simulink model "VMC_14Dof_2024a"  (R2024a)
settings: Solver=FixedStepDiscrete  StartTime=0.0  StopTime=10.0  FixedStep=0.001  RelTol=1e-3
InitFcn:
  | unlinear_14DOF_Parameters
undefined symbols (not defined in the file): Bf, Br, Cp_fl, Cp_fr, Cp_rl, Cp_rr, Cs_f, eta_FMotor, eta_RMotor, f, g, He, Hp, i_fa, i_ra, i_sw, I_tire, Ix, Iy, Iz, ks_f, kw, Lf, Lr, m, mb, mu, mw, r, Sampletime, Standstill_buffer, vx0, vxlim, w0
libraries: simulink x32, slpidlib x6
(part 3 of 5)

== system VMC_14Dof_2024a/Subsystem1/Vehicle_State_Estimation/Steering_Angle ==
  SteeringWheelAngle_deg : Inport
  Constant3 : Constant  Value=0  OutDataTypeStr=single  SampleTime=-1
  Constant4 : Constant  Value=0  OutDataTypeStr=single  SampleTime=-1
  FWA_FL_Table_deg : Lookup_n-D  NumberOfTableDimensions=1  BreakpointsForDimension1=|  BreakpointsForDimension1DataTypeStr=single  Table=|  TableDataTypeStr=single  IntermediateResultsDataTypeStr=single  InternalRulePriority=Speed  OutDataTypeStr=single  RndMeth=Simplest  FractionDataTypeStr=single
      BreakpointsForDimension1=|
      | [-117
      | -116
      | -115
      | -114
      | -113
      | -112
      | -111
      | -110
      | -109
      | -108
      | -107
      | -106
      | -105
      | -104
      | -103
      | -102
      | -101
      | -100
      | -99
      | -98
      | -97
      | -96
      | -95
      | -94
      | -93
      | -92
      | -91
      | -90
      | -89
      | -88
      | -87
      | -86
      | -85
      | -84
      | -83
      | -82
      | -81
      | -80
      | -79
      | -78
      | -77
      | -76
      | -75
      | -74
      | -73
      | -72
      | -71
      | -70
      | -69
      | -68
      | -67
      | -66
      | -65
      | -64
      | -63
      | -62
      | -61
      | -60
      | -59
      | -58
      | -57
      | -56
      | -55
      | -54
      | -53
      | -52
      | -51
      | -50
      | -49
      | -48
      | -47
      | -46
      | -45
      | -44
      | -43
      | -42
      | -41
      | -40
      | -39
      | -38
      | -37
      | -36
      | -35
      | -34
      | -33
      | -32
      | -31
      | -30
      | -29
      | -28
      | -27
      | -26
      | -25
      | -24
      | -23
      | -22
      | -21
      | -20
      | -19
      | -18
      | -17
      | -16
      | -15
      | -14
      | -13
      | -12
      | -11
      | -10
      | -9
      | -8
      | -7
      | -6
      | -5
      | -4
      | -3
      | -2
      | -1
      | 0
      | 1
      | 2
      | 3
      | 4
      | 5
      | 6
      | 7
      | 8
      | 9
      | 10
      | 11
      | 12
      | 13
      | 14
      | 15
      | 16
      | 17
      | 18
      | 19
      | 20
      | 21
      | 22
      | 23
      | 24
      | 25
      | 26
      | 27
      | 28
      | 29
      | 30
      | 31
      | 32
      | 33
      | 34
      | 35
      | 36
      | 37
      | 38
      | 39
      | 40
      | 41
      | 42
      | 43
      | 44
      | 45
      | 46
      | 47
      | 48
      | 49
      | 50
      | 51
      | 52
      | 53
      | 54
      | 55
      | 56
      | 57
      | 58
      | 59
      | 60
      | 61
      | 62
      | 63
      | 64
      | 65
      | 66
      | 67
      | 68
      | 69
      | 70
      | 71
      | 72
      | 73
      | 74
      | 75
      | 76
      | 77
      | 78
      | 79
      | 80
      | 81
      | 82
      | 83
      | 84
      | 85
      | 86
      | 87
      | 88
      | 89
      | 90
      | 91
      | 92
      | 93
      | 94
      | 95
      | 96
      | 97
      | 98
      | 99
      | 100
      | 101
      | 102
      | 103
      | 104
      | 105
      | 106
      | 107
      | 108
      | 109
      | 110
      | 111
      | 112
      | 113
      | 114
      | 115
      | 116
      | 117]
      Table=|
      | [-23.05316527
      | -22.85986982
      | -22.66659264
      | -22.47333151
      | -22.28008425
      | -22.08684866
      | -21.89362256
      | -21.70040379
      | -21.50719018
      | -21.31397955
      | -21.12076975
      | -20.92755864
      | -20.73434405
      | -20.54112386
      | -20.34789591
      | -20.15465809
      | -19.96140824
      | -19.76814426
      | -19.57486401
      | -19.38156538
      | -19.18824624
      | -18.99490448
      | -18.801538
      | -18.60814467
      | -18.4147224
      | -18.22126908
      | -18.0277826
      | -17.83426085
      | -17.64070175
      | -17.44710317
      | -17.25346304
      | -17.05977924
      | -16.86604968
      | -16.67227225
      | -16.47844486
      | -16.2845654
      | -16.09063178
      | -15.89664189
      | -15.70259363
      | -15.5084849
      | -15.31431358
      | -15.12007757
      | -14.92577477
      | -14.73140306
      | -14.53696032
      | -14.34244444
      | -14.14785329
      | -13.95318476
      | -13.75843671
      | -13.56360702
      | -13.36869356
      | -13.17369417
      | -12.97860673
      | -12.78342908
      | -12.58815908
      | -12.39279455
      | -12.19733335
      | -12.00177331
      | -11.80611224
      | -11.61034798
      | -11.41447833
      | -11.2185011
      | -11.0224141
      | -10.82621511
      | -10.62990193
      | -10.43347233
      | -10.23692409
      | -10.04025496
      | -9.843462713
      | -9.646545082
      | -9.449499809
      | -9.252324623
      | -9.055017243
      | -8.857575379
      | -8.659996732
      | -8.46227899
      | -8.264419833
      | -8.066416931
      | -7.868267939
      | -7.669970506
      | -7.471522265
      | -7.27292084
      | -7.07416384
      | -6.875248864
      | -6.676173498
      | -6.476935313
      | -6.277531868
      | -6.077960708
      | -5.878219363
      | -5.678305351
      | -5.478216172
      | -5.277949314
      | -5.077502247
      | -4.876872426
      | -4.676057291
      | -4.475054264
      | -4.273860752
      | -4.072474141
      | -3.870891803
      | -3.669111092
      | -3.467129341
      | -3.264943865
      | -3.062551963
      | -2.859950909
      | -2.657137961
      | -2.454110356
      | -2.250865308
      | -2.047400013
      | -1.843711642
      | -1.639797346
      | -1.435654252
      | -1.231279465
      | -1.026670065
      | -0.82182311
      | -0.616735632
      | -0.411404637
      | -0.205827108
      | 0
      | 0.206079759
      | 0.412415266
      | 0.619009648
      | 0.825866059
      | 1.032987682
      | 1.240377731
      | 1.448039447
      | 1.655976105
      | 1.864191008
      | 2.072687493
      | 2.28146893
      | 2.49053872
      | 2.6999003
      | 2.909557141
      | 3.119512748
      | 3.329770663
      | 3.540334465
      | 3.75120777
      | 3.962394233
      | 4.173897546
      | 4.385721443
      | 4.597869697
      | 4.810346123
      | 5.02315458
      | 5.236298967
      | 5.449783228
      | 5.663611355
      | 5.877787381
      | 6.09231539
      | 6.307199511
      | 6.522443924
      | 6.738052856
      | 6.954030589
      | 7.170381452
      | 7.387109832
      | 7.604220167
      | 7.821716951
      | 8.039604735
      | 8.257888127
      | 8.476571794
      | 8.695660466
      | 8.915158929
      | 9.135072038
      | 9.355404708
      | 9.576161921
      | 9.797348726
      | 10.01897024
      | 10.24103166
      | 10.46353823
      | 10.68649529
      | 10.90990825
      | 11.1337826
      | 11.35812389
      | 11.58293777
      | 11.80822996
      | 12.03400628
      | 12.26027261
      | 12.48703495
      | 12.71429936
      | 12.94207201
      | 13.17035916
      | 13.39916716
      | 13.62850247
      | 13.85837164
      | 14.08878133
      | 14.3197383
      | 14.55124944
      | 14.78332172
      | 15.01596225
      | 15.24917823
      | 15.48297702
      | 15.71736605
      | 15.95235293
      | 16.18794536
      | 16.42415119
      | 16.66097841
      | 16.89843513
      | 17.13652963
      | 17.3752703
      | 17.61466573
      | 17.85472462
      | 18.09545586
      | 18.33686848
      | 18.5789717
      | 18.82177488
      | 19.06528761
      | 19.3095196
      | 19.55448079
      | 19.80018131
      | 20.04663146
      | 20.29384178
      | 20.54182299
      | 20.79058604
      | 21.0401421
      | 21.29050257
      | 21.54167908
      | 21.79368351
      | 22.04652799
      | 22.3002249
      | 22.55478688
      | 22.81022687
      | 23.06655806
      | 23.32379396
      | 23.58194836
      | 23.84103537
      | 24.10106942
      | 24.36206527
      | 24.62403801
      | 24.88700311
      | 25.15097637
      | 25.415974
      | 25.68201259
      | 25.94910911
      | 26.217281
      | 26.48654607
      | 26.75692263
      | 27.02842943
      | ]
  FWA_FR_Table_deg : Lookup_n-D  NumberOfTableDimensions=1  BreakpointsForDimension1=|  BreakpointsForDimension1DataTypeStr=single  Table=|  TableDataTypeStr=single  IntermediateResultsDataTypeStr=single  InternalRulePriority=Speed  OutDataTypeStr=single  RndMeth=Simplest  FractionDataTypeStr=single
      BreakpointsForDimension1=|
      | [-117
      | -116
      | -115
      | -114
      | -113
      | -112
      | -111
      | -110
      | -109
      | -108
      | -107
      | -106
      | -105
      | -104
      | -103
      | -102
      | -101
      | -100
      | -99
      | -98
      | -97
      | -96
      | -95
      | -94
      | -93
      | -92
      | -91
      | -90
      | -89
      | -88
      | -87
      | -86
      | -85
      | -84
      | -83
      | -82
      | -81
      | -80
      | -79
      | -78
      | -77
      | -76
      | -75
      | -74
      | -73
      | -72
      | -71
      | -70
      | -69
      | -68
      | -67
      | -66
      | -65
      | -64
      | -63
      | -62
      | -61
      | -60
      | -59
      | -58
      | -57
      | -56
      | -55
      | -54
      | -53
      | -52
      | -51
      | -50
      | -49
      | -48
      | -47
      | -46
      | -45
      | -44
      | -43
      | -42
      | -41
      | -40
      | -39
      | -38
      | -37
      | -36
      | -35
      | -34
      | -33
      | -32
      | -31
      | -30
      | -29
      | -28
      | -27
      | -26
      | -25
      | -24
      | -23
      | -22
      | -21
      | -20
      | -19
      | -18
      | -17
      | -16
      | -15
      | -14
      | -13
      | -12
      | -11
      | -10
      | -9
      | -8
      | -7
      | -6
      | -5
      | -4
      | -3
      | -2
      | -1
      | 0
      | 1
      | 2
      | 3
      | 4
      | 5
      | 6
      | 7
      | 8
      | 9
      | 10
      | 11
      | 12
      | 13
      | 14
      | 15
      | 16
      | 17
      | 18
      | 19
      | 20
      | 21
      | 22
      | 23
      | 24
      | 25
      | 26
      | 27
      | 28
      | 29
      | 30
      | 31
      | 32
      | 33
      | 34
      | 35
      | 36
      | 37
      | 38
      | 39
      | 40
      | 41
      | 42
      | 43
      | 44
      | 45
      | 46
      | 47
      | 48
      | 49
      | 50
      | 51
      | 52
      | 53
      | 54
      | 55
      | 56
      | 57
      | 58
      | 59
      | 60
      | 61
      | 62
      | 63
      | 64
      | 65
      | 66
      | 67
      | 68
      | 69
      | 70
      | 71
      | 72
      | 73
      | 74
      | 75
      | 76
      | 77
      | 78
      | 79
      | 80
      | 81
      | 82
      | 83
      | 84
      | 85
      | 86
      | 87
      | 88
      | 89
      | 90
      | 91
      | 92
      | 93
      | 94
      | 95
      | 96
      | 97
      | 98
      | 99
      | 100
      | 101
      | 102
      | 103
      | 104
      | 105
      | 106
      | 107
      | 108
      | 109
      | 110
      | 111
      | 112
      | 113
      | 114
      | 115
      | 116
      | 117]
      Table=|
      | [-27.02842943
      | -26.75692263
      | -26.48654607
      | -26.217281
      | -25.94910911
      | -25.68201259
      | -25.415974
      | -25.15097637
      | -24.88700311
      | -24.62403801
      | -24.36206527
      | -24.10106942
      | -23.84103537
      | -23.58194836
      | -23.32379396
      | -23.06655806
      | -22.81022687
      | -22.55478688
      | -22.3002249
      | -22.04652799
      | -21.79368351
      | -21.54167908
      | -21.29050257
      | -21.0401421
      | -20.79058604
      | -20.54182299
      | -20.29384178
      | -20.04663146
      | -19.80018131
      | -19.55448079
      | -19.3095196
      | -19.06528761
      | -18.82177488
      | -18.5789717
      | -18.33686848
      | -18.09545586
      | -17.85472462
      | -17.61466573
      | -17.3752703
      | -17.13652963
      | -16.89843513
      | -16.66097841
      | -16.42415119
      | -16.18794536
      | -15.95235293
      | -15.71736605
      | -15.48297702
      | -15.24917823
      | -15.01596225
      | -14.78332172
      | -14.55124944
      | -14.3197383
      | -14.08878133
      | -13.85837164
      | -13.62850247
      | -13.39916716
      | -13.17035916
      | -12.94207201
      | -12.71429936
      | -12.48703495
      | -12.26027261
      | -12.03400628
      | -11.80822996
      | -11.58293777
      | -11.35812389
      | -11.1337826
      | -10.90990825
      | -10.68649529
      | -10.46353823
      | -10.24103166
      | -10.01897024
      | -9.797348726
      | -9.576161921
      | -9.355404708
      | -9.135072038
      | -8.915158929
      | -8.695660466
      | -8.476571794
      | -8.257888127
      | -8.039604735
      | -7.821716951
      | -7.604220167
      | -7.387109832
      | -7.170381452
      | -6.954030589
      | -6.738052856
      | -6.522443924
      | -6.307199511
      | -6.09231539
      | -5.877787381
      | -5.663611355
      | -5.449783228
      | -5.236298967
      | -5.02315458
      | -4.810346123
      | -4.597869697
      | -4.385721443
      | -4.173897546
      | -3.962394233
      | -3.75120777
      | -3.540334465
      | -3.329770663
      | -3.119512748
      | -2.909557141
      | -2.6999003
      | -2.49053872
      | -2.28146893
      | -2.072687493
      | -1.864191008
      | -1.655976105
      | -1.448039447
      | -1.240377731
      | -1.032987682
      | -0.825866059
      | -0.619009648
      | -0.412415266
      | -0.206079759
      | 0
      | 0.205827108
      | 0.411404637
      | 0.616735632
      | 0.82182311
      | 1.026670065
      | 1.231279465
      | 1.435654252
      | 1.639797346
      | 1.843711642
      | 2.047400013
      | 2.250865308
      | 2.454110356
      | 2.657137961
      | 2.859950909
      | 3.062551963
      | 3.264943865
      | 3.467129341
      | 3.669111092
      | 3.870891803
      | 4.072474141
      | 4.273860752
      | 4.475054264
      | 4.676057291
      | 4.876872426
      | 5.077502247
      | 5.277949314
      | 5.478216172
      | 5.678305351
      | 5.878219363
      | 6.077960708
      | 6.277531868
      | 6.476935313
      | 6.676173498
      | 6.875248864
      | 7.07416384
      | 7.27292084
      | 7.471522265
      | 7.669970506
      | 7.868267939
      | 8.066416931
      | 8.264419833
      | 8.46227899
      | 8.659996732
      | 8.857575379
      | 9.055017243
      | 9.252324623
      | 9.449499809
      | 9.646545082
      | 9.843462713
      | 10.04025496
      | 10.23692409
      | 10.43347233
      | 10.62990193
      | 10.82621511
      | 11.0224141
      | 11.2185011
      | 11.41447833
      | 11.61034798
      | 11.80611224
      | 12.00177331
      | 12.19733335
      | 12.39279455
      | 12.58815908
      | 12.78342908
      | 12.97860673
      | 13.17369417
      | 13.36869356
      | 13.56360702
      | 13.75843671
      | 13.95318476
      | 14.14785329
      | 14.34244444
      | 14.53696032
      | 14.73140306
      | 14.92577477
      | 15.12007757
      | 15.31431358
      | 15.5084849
      | 15.70259363
      | 15.89664189
      | 16.09063178
      | 16.2845654
      | 16.47844486
      | 16.67227225
      | 16.86604968
      | 17.05977924
      | 17.25346304
      | 17.44710317
      | 17.64070175
      | 17.83426085
      | 18.0277826
      | 18.22126908
      | 18.4147224
      | 18.60814467
      | 18.801538
      | 18.99490448
      | 19.18824624
      | 19.38156538
      | 19.57486401
      | 19.76814426
      | 19.96140824
      | 20.15465809
      | 20.34789591
      | 20.54112386
      | 20.73434405
      | 20.92755864
      | 21.12076975
      | 21.31397955
      | 21.50719018
      | 21.70040379
      | 21.89362256
      | 22.08684866
      | 22.28008425
      | 22.47333151
      | 22.66659264
      | 22.85986982
      | 23.05316527
      | ]
  Gain6 : Gain  Gain=pi/180  OutDataTypeStr=single
  Gain7 : Gain  Gain=pi/180  OutDataTypeStr=single
  Mux : Mux
  Saturation : Saturate  UpperLimit=117  LowerLimit=-117  OutDataTypeStr=single
  WheelAngle_Array_rad : Outport
  wires:
  FWA_FL_Table_deg/1 -> Gain6/1
  Gain6/1 -> Mux/1  "Steering_Angle_ByRad"
  Mux/1 -> WheelAngle_Array_rad/1
  Constant3/1 -> Mux/3  "RL_Wheel_Angle"
  FWA_FR_Table_deg/1 -> Gain7/1
  Gain7/1 -> Mux/2  "Steering_Angle_ByRad"
  Constant4/1 -> Mux/4  "RR_Wheel_Angle"
  Saturation/1 -> FWA_FR_Table_deg/1, FWA_FL_Table_deg/1
  SteeringWheelAngle_deg/1 -> Saturation/1

== system VMC_14Dof_2024a/Subsystem1/Vehicle_State_Estimation/Tire_Force ==
  m_FL_kg : Inport
  m_FR_kg : Inport  Port=2
  m_RL_kg : Inport  Port=3
  m_RR_kg : Inport  Port=4
  ax_mpss : Inport  Port=5
  ay_mpss : Inport  Port=6
  h_CoG_m : Inport  Port=7
  Wheelbase_m : Inport  Port=8
  Krf_Nmprad : Inport  Port=9
  Krr_Nmprad : Inport  Port=10
  Zrf_m : Inport  Port=11
  Zrr_m : Inport  Port=12
  tf_m : Inport  Port=13
  tr_m : Inport  Port=14
  lf_m : Inport  Port=15
  lr_m : Inport  Port=16
  ClA : Inport  Port=17
  rho : Inport  Port=18
  V_CoG_mps : Inport  Port=19
  Aero_Ratio : Inport  Port=20
  Mux : Mux
  Normal_Force : Subsystem
  Fz_Array_N : Outport
  wires:
  Normal_Force/1(Fz_FL_N) -> Mux/1
  Normal_Force/2(Fz_FR_N) -> Mux/2
  Normal_Force/3(Fz_RL_N) -> Mux/3
  Normal_Force/4(Fz_RR_N) -> Mux/4
  Mux/1 -> Fz_Array_N/1
  m_FL_kg/1 -> Normal_Force/1(m_FL_kg)
  m_FR_kg/1 -> Normal_Force/2(m_FR_kg)
  m_RL_kg/1 -> Normal_Force/3(m_RL_kg)
  m_RR_kg/1 -> Normal_Force/4(m_RR_kg)
  ax_mpss/1 -> Normal_Force/5(ax_mpss)
  ay_mpss/1 -> Normal_Force/6(ay_mpss)
  h_CoG_m/1 -> Normal_Force/7(h_CoG_m)
  Wheelbase_m/1 -> Normal_Force/8(Wheelbase_m)
  Krf_Nmprad/1 -> Normal_Force/9(Krf_Nmprad)
  Krr_Nmprad/1 -> Normal_Force/10(Krr_Nmprad)
  Zrf_m/1 -> Normal_Force/11(Zrf_m)
  Zrr_m/1 -> Normal_Force/12(Zrr_m)
  tf_m/1 -> Normal_Force/13(tf_m)
  tr_m/1 -> Normal_Force/14(tr_m)
  lf_m/1 -> Normal_Force/15(lf_m)
  lr_m/1 -> Normal_Force/16(lr_m)
  ClA/1 -> Normal_Force/17(ClA)
  rho/1 -> Normal_Force/18(rho)
  V_CoG_mps/1 -> Normal_Force/19(V_CoG_mps)
  Aero_Ratio/1 -> Normal_Force/20(Aero_Ratio)

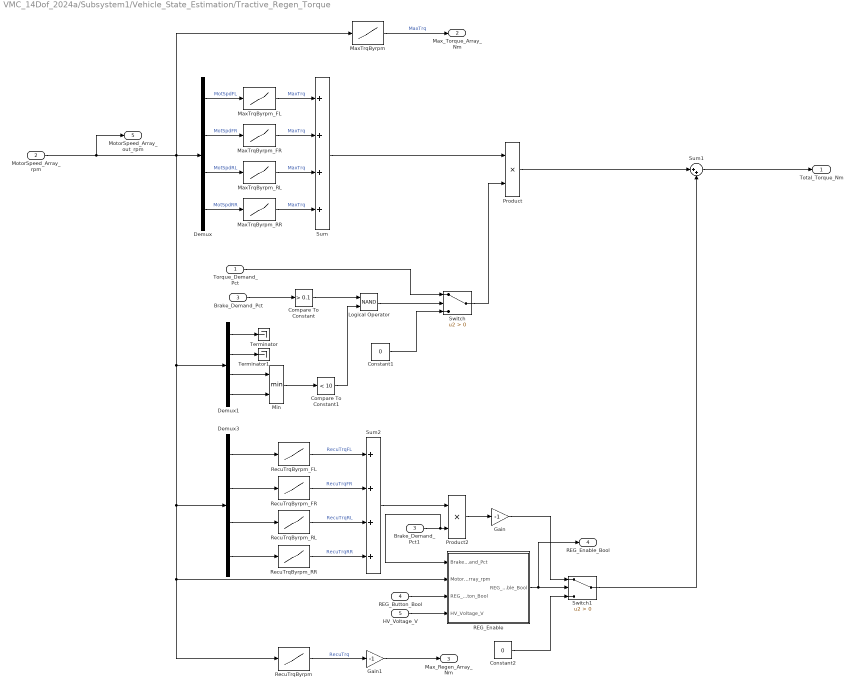
== system VMC_14Dof_2024a/Subsystem1/Vehicle_State_Estimation/Tractive_Regen_Torque ==
  Torque_Demand_Pct : Inport  OutDataTypeStr=single
  MotorSpeed_Array_rpm : Inport  Port=2  OutDataTypeStr=single
  Brake_Demand_Pct : Inport  Port=3  OutDataTypeStr=single
  REG_Button_Bool : Inport  Port=4
  HV_Voltage_V : Inport  Port=5
  Brake_Demand_Pct1 : InportShadow  Port=3  OutDataTypeStr=single
  Compare To Constant : simulink/Logic and Bit Operations/Compare To Constant  relop=>  const=0.1  OutDataTypeStr=boolean
  Compare To Constant1 : simulink/Logic and Bit Operations/Compare To Constant  relop=<  const=10  OutDataTypeStr=boolean
  Constant1 : Constant  Value=0  OutDataTypeStr=single  SampleTime=-1
  Constant2 : Constant  Value=0  OutDataTypeStr=single  SampleTime=-1
  Demux : Demux
  Demux1 : Demux
  Demux3 : Demux
  Gain : Gain  Gain=-1  ParamDataTypeStr=single  OutDataTypeStr=single
  Gain1 : Gain  Gain=-1  ParamDataTypeStr=single  OutDataTypeStr=single
  Logical Operator : Logic  Operator=NAND  AllPortsSameDT=off  OutDataTypeStr=boolean
  MaxTrqByrpm : Lookup_n-D  NumberOfTableDimensions=1  BreakpointsForDimension1=[0,16000,19999,20000]  BreakpointsForDimension1DataTypeStr=single  Table=[21,21,13,0]  TableDataTypeStr=single  IntermediateResultsDataTypeStr=single  InternalRulePriority=Speed  OutDataTypeStr=single  RndMeth=Simplest  FractionDataTypeStr=single
  MaxTrqByrpm_FL : Lookup_n-D  NumberOfTableDimensions=1  BreakpointsForDimension1=[0,16000,19999,20000]  BreakpointsForDimension1DataTypeStr=single  Table=[21,21,13,0]  TableDataTypeStr=single  IntermediateResultsDataTypeStr=single  InternalRulePriority=Speed  OutDataTypeStr=single  RndMeth=Simplest  FractionDataTypeStr=single
  MaxTrqByrpm_FR : Lookup_n-D  NumberOfTableDimensions=1  BreakpointsForDimension1=[0,16000,19999,20000]  BreakpointsForDimension1DataTypeStr=single  Table=[21,21,13,0]  TableDataTypeStr=single  IntermediateResultsDataTypeStr=single  InternalRulePriority=Speed  OutDataTypeStr=single  RndMeth=Simplest  FractionDataTypeStr=single
  MaxTrqByrpm_RL : Lookup_n-D  NumberOfTableDimensions=1  BreakpointsForDimension1=[0,16000,19999,20000]  BreakpointsForDimension1DataTypeStr=single  Table=[21,21,13,0]  TableDataTypeStr=single  IntermediateResultsDataTypeStr=single  InternalRulePriority=Speed  OutDataTypeStr=single  RndMeth=Simplest  FractionDataTypeStr=single
  MaxTrqByrpm_RR : Lookup_n-D  NumberOfTableDimensions=1  BreakpointsForDimension1=[0,16000,19999,20000]  BreakpointsForDimension1DataTypeStr=single  Table=[21,21,13,0]  TableDataTypeStr=single  IntermediateResultsDataTypeStr=single  InternalRulePriority=Speed  OutDataTypeStr=single  RndMeth=Simplest  FractionDataTypeStr=single
  Min : MinMax  Inputs=2
  Product : Product
  Product2 : Product  OutDataTypeStr=single
  REG_Enable : Subsystem
  RecuTrqByrpm : Lookup_n-D  NumberOfTableDimensions=1  BreakpointsForDimension1=[0,1500,5000,20000]  BreakpointsForDimension1DataTypeStr=single  Table=[0,0,17,17]  TableDataTypeStr=single  IntermediateResultsDataTypeStr=single  InternalRulePriority=Speed  OutDataTypeStr=single  RndMeth=Simplest  FractionDataTypeStr=single
  RecuTrqByrpm_FL : Lookup_n-D  NumberOfTableDimensions=1  BreakpointsForDimension1=[0,1500,5000,20000]  BreakpointsForDimension1DataTypeStr=single  Table=[0,0,17,17]  TableDataTypeStr=single  IntermediateResultsDataTypeStr=single  InternalRulePriority=Speed  OutDataTypeStr=single  RndMeth=Simplest  FractionDataTypeStr=single
  RecuTrqByrpm_FR : Lookup_n-D  NumberOfTableDimensions=1  BreakpointsForDimension1=[0,1500,5000,20000]  BreakpointsForDimension1DataTypeStr=single  Table=[0,0,17,17]  TableDataTypeStr=single  IntermediateResultsDataTypeStr=single  InternalRulePriority=Speed  OutDataTypeStr=single  RndMeth=Simplest  FractionDataTypeStr=single
  RecuTrqByrpm_RL : Lookup_n-D  NumberOfTableDimensions=1  BreakpointsForDimension1=[0,1500,5000,20000]  BreakpointsForDimension1DataTypeStr=single  Table=[0,0,17,17]  TableDataTypeStr=single  IntermediateResultsDataTypeStr=single  InternalRulePriority=Speed  OutDataTypeStr=single  RndMeth=Simplest  FractionDataTypeStr=single
  RecuTrqByrpm_RR : Lookup_n-D  NumberOfTableDimensions=1  BreakpointsForDimension1=[0,1500,5000,20000]  BreakpointsForDimension1DataTypeStr=single  Table=[0,0,17,17]  TableDataTypeStr=single  IntermediateResultsDataTypeStr=single  InternalRulePriority=Speed  OutDataTypeStr=single  RndMeth=Simplest  FractionDataTypeStr=single
  Sum : Sum  Inputs=++++
  Sum1 : Sum  Inputs=|++  OutDataTypeStr=single  AccumDataTypeStr=single
  Sum2 : Sum  Inputs=++++  AccumDataTypeStr=single
  Switch : Switch  Criteria=u2 > Threshold  OutDataTypeStr=single  SaturateOnIntegerOverflow=off  InputSameDT=off
  Switch1 : Switch  Criteria=u2 > Threshold  OutDataTypeStr=single  SaturateOnIntegerOverflow=off  InputSameDT=off
  Terminator : Terminator
  Terminator1 : Terminator
  Total_Torque_Nm : Outport
  Max_Torque_Array_Nm : Outport  Port=2
  Max_Regen_Array_Nm : Outport  Port=3
  REG_Enable_Bool : Outport  Port=4
  MotorSpeed_Array_out_rpm : Outport  Port=5
  wires:
  Demux/1 -> MaxTrqByrpm_FL/1  "MotSpdFL"
  Demux/2 -> MaxTrqByrpm_FR/1  "MotSpdFR"
  Demux/3 -> MaxTrqByrpm_RL/1  "MotSpdRL"
  Demux/4 -> MaxTrqByrpm_RR/1  "MotSpdRR"
  MaxTrqByrpm_FL/1 -> Sum/1  "MaxTrq"
  MaxTrqByrpm_FR/1 -> Sum/2  "MaxTrq"
  MaxTrqByrpm_RL/1 -> Sum/3  "MaxTrq"
  MaxTrqByrpm_RR/1 -> Sum/4  "MaxTrq"
  Sum/1 -> Product/1
  MaxTrqByrpm/1 -> Max_Torque_Array_Nm/1  "MaxTrq"
  Demux1/2 -> Terminator1/1
  Demux1/3 -> Min/1
  Switch/1 -> Product/2
  Constant1/1 -> Switch/3
  Logical Operator/1 -> Switch/2
  Demux1/4 -> Min/2
  Compare To Constant/1 -> Logical Operator/1
  Min/1 -> Compare To Constant1/1
  Demux1/1 -> Terminator/1
  Compare To Constant1/1 -> Logical Operator/2
  MotorSpeed_Array_rpm/1 -> MotorSpeed_Array_out_rpm/1, Demux1/1, RecuTrqByrpm/1, REG_Enable/2(MotorSpeed_Array_rpm), Demux3/1, MaxTrqByrpm/1, Demux/1
  Torque_Demand_Pct/1 -> Switch/1
  Brake_Demand_Pct/1 -> Compare To Constant/1
  REG_Enable/1(REG_Enable_Bool) -> REG_Enable_Bool/1, Switch1/2
  Gain/1 -> Switch1/1
  Brake_Demand_Pct1/1 -> REG_Enable/1(Brake_Demand_Pct), Product2/2
  Demux3/2 -> RecuTrqByrpm_FR/1
  Demux3/3 -> RecuTrqByrpm_RL/1
  Demux3/1 -> RecuTrqByrpm_FL/1
  Sum2/1 -> Product2/1
  Product2/1 -> Gain/1
  RecuTrqByrpm_RL/1 -> Sum2/3  "RecuTrqRL"
  RecuTrqByrpm_FL/1 -> Sum2/1  "RecuTrqFL"
  RecuTrqByrpm_FR/1 -> Sum2/2  "RecuTrqFR"
  Demux3/4 -> RecuTrqByrpm_RR/1
  RecuTrqByrpm_RR/1 -> Sum2/4  "RecuTrqRR"
  Constant2/1 -> Switch1/3
  REG_Button_Bool/1 -> REG_Enable/3(REG_Button_Bool)
  HV_Voltage_V/1 -> REG_Enable/4(HV_Voltage_V)
  Product/1 -> Sum1/1
  Sum1/1 -> Total_Torque_Nm/1
  Switch1/1 -> Sum1/2
  RecuTrqByrpm/1 -> Gain1/1  "RecuTrq"
  Gain1/1 -> Max_Regen_Array_Nm/1

== system VMC_14Dof_2024a/Subsystem1/Vehicle_State_Estimation/Velocity_Estimation ==
  IMU_YawRate_radps : Inport
  OS_Vx_kph : Inport  Port=2
  OS_Vy_kph : Inport  Port=3
  OS_X_Distance_m : Inport  Port=4
  OS_Y_Distance_m : Inport  Port=5
  CoG_Linear_Velocity_Calculation : MATLAB Function  TreatAsAtomicUnit=on
  CoG_Vx_mps : Outport
  CoG_Vy_mps : Outport  Port=2
  CoG_V_mps : Outport  Port=3
  OS_V_mps : Outport  Port=4
  wires:
  IMU_YawRate_radps/1 -> CoG_Linear_Velocity_Calculation/1(Actual_Yaw_Rate)
  OS_Vx_kph/1 -> CoG_Linear_Velocity_Calculation/2(OS_Vx)
  OS_Vy_kph/1 -> CoG_Linear_Velocity_Calculation/3(OS_Vy)
  OS_X_Distance_m/1 -> CoG_Linear_Velocity_Calculation/4(OS_X_Distance)
  OS_Y_Distance_m/1 -> CoG_Linear_Velocity_Calculation/5(OS_Y_Distance)
  CoG_Linear_Velocity_Calculation/1(CoG_Vx) -> CoG_Vx_mps/1
  CoG_Linear_Velocity_Calculation/2(CoG_Vy) -> CoG_Vy_mps/1
  CoG_Linear_Velocity_Calculation/3(CoG_V) -> CoG_V_mps/1
  CoG_Linear_Velocity_Calculation/4(OS_V) -> OS_V_mps/1

== system VMC_14Dof_2024a/Subsystem1/Vehicle_State_Estimation/Wheel_State ==
  GearRatio_NA : Inport
  MotorSpeed_Array_rpm : Inport  Port=2  PortDimensions=[4,1]
  CoG_vx_mps : Inport  Port=3
  CoG_vy_mps : Inport  Port=4
  Yawrate_radps : Inport  Port=5
  WheelAngle_Array_rad : Inport  Port=6  PortDimensions=[4,1]
  lf_m : Inport  Port=7
  lr_m : Inport  Port=8
  Trackwidth_Front_m : Inport  Port=9
  Trackwidth_Rear_m : Inport  Port=10
  Offset_CoG_y_m : Inport  Port=11
  Rolling_Radius_m : Inport  Port=12
  Gain : Gain  Gain=0.5
  Gain1 : Gain  Gain=0.5
  Mux : Mux
  Mux1 : Mux
  Mux2 : Mux  Inputs=2
  Mux3 : Mux
  Mux4 : Mux  Inputs=2
  SlipRatioCal : MATLAB Function  TreatAsAtomicUnit=on
  WhlSpdActlCal : MATLAB Function  TreatAsAtomicUnit=on
  WhlSpdLongCal : MATLAB Function  TreatAsAtomicUnit=on
  WhlSpdRefsCal : MATLAB Function  TreatAsAtomicUnit=on
  Act_WheelSpeed_Array_radps : Outport
  Ref_WheelSpeed_Array_radps : Outport  Port=2
  SlipRatio_Array_NA : Outport  Port=3
  Tire_SlipAngle_Array_rad : Outport  Port=4
  wires:
  MotorSpeed_Array_rpm/1 -> WhlSpdActlCal/2(MotSpdByrpm)
  GearRatio_NA/1 -> WhlSpdActlCal/1(Gear_Ratio)
  WhlSpdActlCal/1(WhlSpdActlFL) -> Mux3/1
  WhlSpdActlCal/2(WhlSpdActlFR) -> Mux3/2
  WhlSpdActlCal/3(WhlSpdActlRL) -> Mux3/3
  WhlSpdActlCal/4(WhlSpdActlRR) -> Mux3/4
  Mux3/1 -> SlipRatioCal/1(Actl), Act_WheelSpeed_Array_radps/1  "WhlSpdActlByM"
  WhlSpdRefsCal/1(WhlSpdRefFL) -> WhlSpdLongCal/1(WhlSpdRefFL)
  WhlSpdRefsCal/2(WhlSpdRefFR) -> WhlSpdLongCal/2(WhlSpdRefFR)
  WhlSpdRefsCal/3(WhlSpdRefRL) -> WhlSpdLongCal/3(WhlSpdRefRL)
  WhlSpdRefsCal/4(WhlSpdRefRR) -> WhlSpdLongCal/4(WhlSpdRefRR)
  WhlSpdLongCal/1(WhlSpdRefFL_Long) -> Mux/1
  WhlSpdLongCal/2(WhlSpdRefFR_Long) -> Mux/2
  WhlSpdLongCal/3(WhlSpdRefRL_Long) -> Mux/3
  WhlSpdLongCal/4(WhlSpdRefRR_Long) -> Mux/4
  WhlSpdLongCal/5(SA_FL) -> Mux1/1
  WhlSpdLongCal/6(SA_FR) -> Mux1/2
  WhlSpdLongCal/7(SA_RL) -> Mux1/3
  WhlSpdLongCal/8(SA_RR) -> Mux1/4
  Mux/1 -> Ref_WheelSpeed_Array_radps/1, SlipRatioCal/2(Ref)
  CoG_vx_mps/1 -> WhlSpdRefsCal/1(CoG_vx)
  CoG_vy_mps/1 -> WhlSpdRefsCal/2(CoG_vy)
  Yawrate_radps/1 -> WhlSpdRefsCal/3(Yawrate)
  WheelAngle_Array_rad/1 -> WhlSpdRefsCal/4(WheelAngle)
  lf_m/1 -> WhlSpdRefsCal/5(lf)
  lr_m/1 -> WhlSpdRefsCal/6(lr)
  Offset_CoG_y_m/1 -> WhlSpdRefsCal/9(Offset_CoG_y)
  Rolling_Radius_m/1 -> WhlSpdLongCal/5(rolling_radius)
  SlipRatioCal/1(SlipRate) -> SlipRatio_Array_NA/1
  Mux1/1 -> Tire_SlipAngle_Array_rad/1
  Mux2/1 -> WhlSpdRefsCal/7(tf)
  Gain/1 -> Mux2/2, Mux2/1
  Trackwidth_Front_m/1 -> Gain/1
  Gain1/1 -> Mux4/1, Mux4/2
  Mux4/1 -> WhlSpdRefsCal/8(tr)
  Trackwidth_Rear_m/1 -> Gain1/1

== system VMC_14Dof_2024a/Subsystem1/YawRate_Controller/CalMz_FB ==
  RefYawRate_radps : Inport
  Vehicle_States : Inport  Port=2
  Controller_Setting : Inport  Port=3
  Avg_Wheel_Angle : Subsystem
  Bus Selector : BusSelector  OutputSignals=IMU.YawRate_radps,WheelAngle.WheelAngle_Array_rad,IMU.Lateral_Acc_mpss,Vehicle_Velocity.CoG_V_mps
  Bus Selector1 : BusSelector  OutputSignals=TV_Controller.TV_PID.TV_P,TV_Controller.TV_PID.TV_I,TV_Controller.TV_PID.TV_D
  Compare To Constant : simulink/Logic and Bit Operations/Compare To Constant  relop=>=  const=5  OutDataTypeStr=boolean
  Constant : Constant  Value=100  OutDataTypeStr=single
  Constant1 : Constant  Value=0  OutDataTypeStr=single
  PID Controller : slpidlib/PID Controller  Controller=PID  Form=Parallel  TimeDomain=Discrete-time  UseExternalTs=off  SampleTime=-1  IntegratorMethod=Forward Euler  FilterMethod=Forward Euler  ControllerParametersSource=external  P=40  I=12  UseKiTs=off  D=0  UseExternalDerivativeSource=off  N=100  UseFilter=on  TunerSelectOption=Transfer Function Based (PID Tuner App)  InitialConditionSource=internal  InitialConditionForIntegrator=0  InitialConditionForFilter=0  DifferentiatorICPrevScaledInput=0  ExternalReset=rising  TrackingMode=off  Kt=1  LimitOutput=off  SatLimitsSource=internal  UpperSaturationLimit=inf  LowerSaturationLimit=-inf  LinearizeAsGain=on  AntiWindupMode=none  Kb=1  LimitIntegrator=off  UpperIntegratorSaturationLimit=inf  LowerIntegratorSaturationLimit=-inf  POutMin=[]  POutMax=[]  IOutMin=[]  IOutMax=[]  DOutMin=[]  DOutMax=[]  NOutMin=[]  NOutMax=[]  SumOutMin=[]  SumOutMax=[]  SaturationOutMin=[]  SaturationOutMax=[]  PParamMin=[]  PParamMax=[]  IParamMin=[]  IParamMax=[]  DParamMin=[]  DParamMax=[]  NParamMin=[]  NParamMax=[]  KbParamMin=[]  KbParamMax=[]  KtParamMin=[]  KtParamMax=[]  KbOutMin=[]  KbOutMax=[]  KtOutMin=[]  KtOutMax=[]  IntegratorOutMin=[]  IntegratorOutMax=[]  FilterOutMin=[]  FilterOutMax=[]  SumI1OutMin=[]  SumI1OutMax=[]  SumI2OutMin=[]  SumI2OutMax=[]  SumI3OutMin=[]  SumI3OutMax=[]  SumI4OutMin=[]  SumI4OutMax=[]  SumDOutMin=[]  SumDOutMax=[]  DifferentiatorOutMin=[]  DifferentiatorOutMax=[]  FilterDiffOutCoefMin=[]  FilterDiffOutCoefMax=[]  ReciprocalOutMin=[]  ReciprocalOutMax=[]  SumDenOutMin=[]  SumDenOutMax=[]  SumNumOutMin=[]  SumNumOutMax=[]  DivideOutMin=[]  DivideOutMax=[]  UdiffTsProdOutMin=[]  UdiffTsProdOutMax=[]  NTsProdOutMin=[]  NTsProdOutMax=[]  UintegralTsProdOutMin=[]  UintegralTsProdOutMax=[]  UngainTsProdOutMin=[]  UngainTsProdOutMax=[]  ClampingZeroOutDataTypeStr=Inherit: Inherit via back propagation  ClampingZeroOutMin=[]  ClampingZeroOutMax=[]  FilterDenConstantOutDataTypeStr=Inherit: Inherit via back propagation  FilterDenConstantOutMin=[]  FilterDenConstantOutMax=[]  PCopyOutDataTypeStr=Inherit: Inherit via back propagation  PCopyOutMin=[]  PCopyOutMax=[]  NCopyOutDataTypeStr=Inherit: Inherit via back propagation  NCopyOutMin=[]  NCopyOutMax=[]  IntegratorContinuousStateAttributes=''  IntegratorStateMustResolveToSignalObject=off  IntegratorRTWStateStorageClass=Auto  FilterContinuousStateAttributes=''  FilterStateMustResolveToSignalObject=off  FilterRTWStateStorageClass=Auto  ParallelPVariant=ExternalParameters  IdealPVariant=Disabled  IVariant=ExternalParameters  DVariant=ExternalParameters  IntegratorVariant=Discrete  SatVariant=Disabled  AWVariant=Passthrough  PCopyVariant=Disabled  TRVariant=Disabled  FdbkBlocksVariant=Forward  IdealPFdbkVariant=Disabled  SatFdbkVariant=Disabled  DerivativeFilterVariant=ForwardEulerFilter  NVariant=ExternalParameters  NCopyVariant=Disabled  FilterICVariant=InternalICsFilter  IntegratorICVariant=InternalICs  ExternalResetVariant=ExternalReset  TRSumVariant=Passthrough  SumFdbkVariant=Disabled  SumVariant=Sum_PID  TsampFilterVariant=InternalTs  TsampNgainVariant=Passthrough  TsampIntegralVariant=Disabled_SignalSpec  ExternalSaturationOutDataTypeStr=Inherit: Same as second input  DerivativeSourceVariant=ErrorSignal
  Rad_To_Degree_Factor : Gain  Gain=180/pi  ParamDataTypeStr=single
  Saturation : Saturate  UpperLimit=1500  LowerLimit=-1500  OutDataTypeStr=single
  Sum : Sum  Inputs=|+-  OutDataTypeStr=single  AccumDataTypeStr=single
  Switch : Switch  Criteria=u2 > Threshold  SaturateOnIntegerOverflow=off  InputSameDT=off
  TV_Reset : Subsystem
  ExtYawMoment_FB : Outport
  YawRateErr_radps : Outport  Port=2
  wires:
  PID Controller/1 -> Saturation/1
  Sum/1 -> Rad_To_Degree_Factor/1, YawRateErr_radps/1
  Rad_To_Degree_Factor/1 -> PID Controller/1
  TV_Reset/1(TV_Reset) -> PID Controller/6
  Bus Selector1/2 -> PID Controller/3  "<TV_I>"
  Bus Selector1/3 -> PID Controller/4  "<TV_D>"
  Bus Selector1/1 -> PID Controller/2  "<TV_P>"
  Constant/1 -> PID Controller/5
  Controller_Setting/1 -> Bus Selector1/1
  RefYawRate_radps/1 -> Sum/1
  Vehicle_States/1 -> Bus Selector/1
  Bus Selector/1 -> Sum/2  "<YawRate_radps>"
  Bus Selector/3 -> TV_Reset/2(LateralAcceleration_mpss)  "<Lateral_Acc_mpss>"
  Avg_Wheel_Angle/1(Avg_WheelAngle_rad) -> TV_Reset/1(Avg_WheelAngle_rad)
  Bus Selector/2 -> Avg_Wheel_Angle/1(WheelAngle_Array_rad)  "<WheelAngle_Array_rad>"
  Saturation/1 -> Switch/1
  Switch/1 -> ExtYawMoment_FB/1
  Constant1/1 -> Switch/3
  Compare To Constant/1 -> Switch/2
  Bus Selector/4 -> Compare To Constant/1  "<CoG_V_mps>"

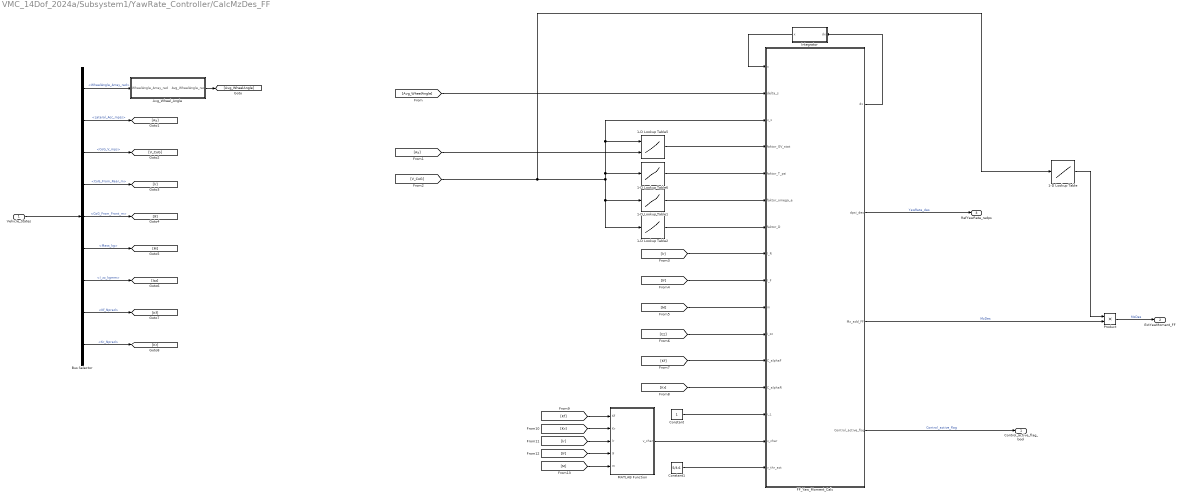
== system VMC_14Dof_2024a/Subsystem1/YawRate_Controller/CalcMzDes_FF ==
  Vehicle_States : Inport
  1-D Lookup Table : Lookup_n-D  NumberOfTableDimensions=1  BreakpointsForDimension1=[0, 5/3.6, 10/3.6, 100]  BreakpointsForDimension1DataTypeStr=single  Table=[0 0 1 1]  TableDataTypeStr=single  IntermediateResultsDataTypeStr=single  InternalRulePriority=Speed  OutDataTypeStr=single  RndMeth=Simplest  FractionDataTypeStr=single
  1-D Lookup Table1 : Lookup_n-D  NumberOfTableDimensions=1  BreakpointsForDimension1=[0, 200]  BreakpointsForDimension1DataTypeStr=single  Table=[1,1]  TableDataTypeStr=single  IntermediateResultsDataTypeStr=single  InternalRulePriority=Speed  OutDataTypeStr=single  RndMeth=Simplest  FractionDataTypeStr=single
  1-D Lookup Table2 : Lookup_n-D  NumberOfTableDimensions=1  BreakpointsForDimension1=[0, 200]  BreakpointsForDimension1DataTypeStr=single  Table=[1,1]  TableDataTypeStr=single  IntermediateResultsDataTypeStr=single  InternalRulePriority=Speed  OutDataTypeStr=single  RndMeth=Simplest  FractionDataTypeStr=single
  1-D Lookup Table5 : Lookup_n-D  BreakpointsForDimension1=[0, 200]  BreakpointsForDimension2=[-20, 20]  BreakpointsForDimension1DataTypeStr=single  BreakpointsForDimension2DataTypeStr=single  Table=[1.1,1.1;1.1,1.1]  TableDataTypeStr=single  IntermediateResultsDataTypeStr=single  InternalRulePriority=Speed  OutDataTypeStr=single  RndMeth=Simplest  FractionDataTypeStr=single
      settings: InputPortMap=u0,u1
  1-D Lookup Table6 : Lookup_n-D  NumberOfTableDimensions=1  BreakpointsForDimension1=[0, 200]  BreakpointsForDimension1DataTypeStr=single  Table=[1,1]  TableDataTypeStr=single  IntermediateResultsDataTypeStr=single  InternalRulePriority=Speed  OutDataTypeStr=single  RndMeth=Simplest  FractionDataTypeStr=single
  Avg_Wheel_Angle : Subsystem
  Bus Selector : BusSelector  OutputSignals=WheelAngle.WheelAngle_Array_rad,IMU.Lateral_Acc_mpss,Vehicle_Velocity.CoG_V_mps,Vehicle_Static_Parameter.CoG_From_Rear_m,Vehicle_Static_Parameter.CoG_From_Front_m,Vehicle_Static_Parameter.Mass_kg,Vehicle_Static_Parameter.I_zz_kgmm,Vehicle_Static_Parameter.Kf_Nprad,Vehicle_Static_Parameter.Kr_Nprad
  Constant : Constant  OutDataTypeStr=single
  Constant1 : Constant  Value=5/3.6  OutDataTypeStr=single
  FF_Yaw_Moment_Calc : MATLAB Function  TreatAsAtomicUnit=on
  Integrator : Subsystem
  MATLAB Function : MATLAB Function  TreatAsAtomicUnit=on
  Product : Product
  Control_active_flag_bool : Outport
  ExtYawMoment_FF : Outport  Port=2
  RefYawRate_radps : Outport  Port=3
  wires:
  Integrator/1(x) -> FF_Yaw_Moment_Calc/1(x)
  [Ay] -> 1-D Lookup Table5/2
  FF_Yaw_Moment_Calc/1(dx) -> Integrator/1(dx)
  FF_Yaw_Moment_Calc/3(Mz_add_FF) -> Product/2  "MzDes"
  FF_Yaw_Moment_Calc/2(dpsi_des) -> RefYawRate_radps/1  "YawRate_des"
  [lr] -> FF_Yaw_Moment_Calc/8(l_R)
  [lf] -> FF_Yaw_Moment_Calc/9(l_F)
  [M] -> FF_Yaw_Moment_Calc/10(m)
  [Izz] -> FF_Yaw_Moment_Calc/11(I_zz)
  [Kf] -> FF_Yaw_Moment_Calc/12(C_alphaF)
  [Kr] -> FF_Yaw_Moment_Calc/13(C_alphaR)
  FF_Yaw_Moment_Calc/4(Control_active_flag) -> Control_active_flag_bool/1  "Control_active_flag"
  [V_CoG] -> 1-D Lookup Table/1, FF_Yaw_Moment_Calc/3(v_x), 1-D Lookup Table5/1, 1-D Lookup Table6/1, 1-D Lookup Table2/1, 1-D Lookup Table1/1
  [Avg_WheelAngle] -> FF_Yaw_Moment_Calc/2(delta_s)
  1-D Lookup Table5/1 -> FF_Yaw_Moment_Calc/4(faktor_GV_stat)
  1-D Lookup Table6/1 -> FF_Yaw_Moment_Calc/5(faktor_T_psi)
  1-D Lookup Table1/1 -> FF_Yaw_Moment_Calc/6(faktor_omega_e)
  1-D Lookup Table2/1 -> FF_Yaw_Moment_Calc/7(faktor_D)
  1-D Lookup Table/1 -> Product/1
  Product/1 -> ExtYawMoment_FF/1  "MzDes"
  Vehicle_States/1 -> Bus Selector/1
  Bus Selector/1 -> Avg_Wheel_Angle/1(WheelAngle_Array_rad)  "<WheelAngle_Array_rad>"
  Avg_Wheel_Angle/1(Avg_WheelAngle_rad) -> [Avg_WheelAngle]
  Bus Selector/2 -> [Ay]  "<Lateral_Acc_mpss>"
  Bus Selector/3 -> [V_CoG]  "<CoG_V_mps>"
  Bus Selector/4 -> [lr]  "<CoG_From_Rear_m>"
  Bus Selector/5 -> [lf]  "<CoG_From_Front_m>"
  Bus Selector/6 -> [M]  "<Mass_kg>"
  Bus Selector/7 -> [Izz]  "<I_zz_kgmm>"
  Bus Selector/8 -> [Kf]  "<Kf_Nprad>"
  Bus Selector/9 -> [Kr]  "<Kr_Nprad>"
  Constant/1 -> FF_Yaw_Moment_Calc/14(i_L)
  MATLAB Function/1(v_char) -> FF_Yaw_Moment_Calc/15(v_char)
  Constant1/1 -> FF_Yaw_Moment_Calc/16(v_thr_act)
  [Kf] -> MATLAB Function/1(Kf)
  [Kr] -> MATLAB Function/2(Kr)
  [lr] -> MATLAB Function/3(lr)
  [lf] -> MATLAB Function/4(lf)
  [M] -> MATLAB Function/5(m)

== system VMC_14Dof_2024a/Subsystem1/YawRate_Controller/Subsystem ==
  ExtYawMoment_FF : Inport
  ExtYawMoment_FB : Inport  Port=2
  YawRateErr_radps : Inport  Port=3
  Controller_Setting : Inport  Port=4
  Bus Selector : BusSelector  OutputSignals=TV_Controller.TV_FF_Enable_bool,TV_Controller.TV_FB_Enable_bool,TV_Controller.TV_ExtMz_Sat_Nm,TV_Controller.TV_ExtMz_Rate_Nmps
  Compare To Constant : simulink/Logic and Bit Operations/Compare To Constant  relop=>  const=0.05  OutDataTypeStr=boolean
  Constant : Constant  Value=0  OutDataTypeStr=single
  Constant1 : Constant  Value=0  OutDataTypeStr=single
  Gain : Gain  Gain=-1
  Gain1 : Gain  Gain=-1
  Logical Operator : Logic  AllPortsSameDT=off  OutDataTypeStr=boolean
  Rate Limiter Dynamic : simulink/Discontinuities/Rate Limiter Dynamic
  Saturation Dynamic : simulink/Discontinuities/Saturation Dynamic  OutMin=[]  OutMax=[]  OutDataTypeStr=Inherit: Same as second input  OutDataType=fixdt(1, 16)  OutScaling=2^-10  DoSatur=off
  Sum : Sum
  Switch : Switch  Criteria=u2 > Threshold  SaturateOnIntegerOverflow=off  InputSameDT=off
  Switch1 : Switch  Criteria=u2 > Threshold  SaturateOnIntegerOverflow=off  InputSameDT=off
  Ext_Mz_Nm : Outport
  wires:
  ExtYawMoment_FF/1 -> Switch/1
  [FF_Control_Flag] -> Switch/2
  Constant/1 -> Switch/3
  ExtYawMoment_FB/1 -> Switch1/1
  YawRateErr_radps/1 -> Compare To Constant/1
  Logical Operator/1 -> Switch1/2
  Compare To Constant/1 -> Logical Operator/1
  [FB_Control_Flag] -> Logical Operator/2
  Constant1/1 -> Switch1/3
  Switch/1 -> Sum/1
  Switch1/1 -> Sum/2
  Sum/1 -> Saturation Dynamic/2
  Rate Limiter Dynamic/1 -> Ext_Mz_Nm/1
  Saturation Dynamic/1 -> Rate Limiter Dynamic/2
  [Ext_Mz_Sat] -> Gain/1, Saturation Dynamic/1
  Gain/1 -> Saturation Dynamic/3
  [Ext_Mz_Rate] -> Gain1/1, Rate Limiter Dynamic/1
  Gain1/1 -> Rate Limiter Dynamic/3
  Controller_Setting/1 -> Bus Selector/1
  Bus Selector/1 -> [FF_Control_Flag]  "<TV_FF_Enable_bool>"
  Bus Selector/2 -> [FB_Control_Flag]  "<TV_FB_Enable_bool>"
  Bus Selector/3 -> [Ext_Mz_Sat]  "<TV_ExtMz_Sat_Nm>"
  Bus Selector/4 -> [Ext_Mz_Rate]  "<TV_ExtMz_Rate_Nmps>"

== system VMC_14Dof_2024a/Subsystem/Body/Suspension_Z/fl ==
  dot_Zs_fl : Inport
  Z_road_fl : Inport  Port=2
  Zs_fl : Inport  Port=3
  . : Gain  Gain=ks_f
  .1 : Gain  Gain=Cs_f
  Add : Sum  Inputs=-+
  Add{1..2,4,6} (4 alike) : Sum  Inputs=+-
  Add3 : Sum
  Add5 : Sum
  Add7 : Sum  OutDataTypeStr=single
  Constant1 : Constant  Value=0.5*mb*g*Lr/(Lf+Lr)  OutDataTypeStr=single
  Constant2 : Constant  Value=0.5*mb*g*Lr/(Lf+Lr)+mw*g  OutDataTypeStr=single
  Gain : Gain  Gain=1/mw
  Gain1 : Gain  Gain=kw
  Gain2 : Gain  Gain=kw
  integrator1 : Subsystem
  integrator2 : Subsystem
  Fzs_fl : Outport  VectorParamsAs1DForOutWhenUnconnected=off
  Fzw_fl : Outport  Port=2  VectorParamsAs1DForOutWhenUnconnected=off
  wires:
  Add5/1 -> Fzs_fl/1
  Constant1/1 -> Add5/2
  integrator1/1(Out) -> integrator2/1(In), Add2/1
  integrator2/1(Out) -> Add6/2, Add1/1, Add/1  "Zw_fl"
  Z_road_fl/1 -> Add/2, Add6/1
  Add/1 -> Gain1/1
  Gain1/1 -> Add4/1  "F2zw_fl"
  Zs_fl/1 -> Add1/2
  Add1/1 -> ./1
  dot_Zs_fl/1 -> Add2/2
  Add2/1 -> .1/1
  ./1 -> Add3/1
  .1/1 -> Add3/2
  Add3/1 -> Add4/2, Add5/1  "F2zs_fl"
  Add4/1 -> Gain/1
  Gain/1 -> integrator1/1(In)
  Add6/1 -> Gain2/1
  Gain2/1 -> Add7/1  "F2zw_fl"
  Constant2/1 -> Add7/2
  Add7/1 -> Fzw_fl/1

== system VMC_14Dof_2024a/Subsystem/Body/Suspension_Z/fr ==
  dot_Zs_fr : Inport
  Z_road_fr : Inport  Port=2
  Zs_fr : Inport  Port=3
  . : Gain  Gain=ks_f
  .1 : Gain  Gain=Cs_f
  Add : Sum  Inputs=-+
  Add{1..2,4,6} (4 alike) : Sum  Inputs=+-
  Add3 : Sum
  Add5 : Sum
  Add7 : Sum  OutDataTypeStr=single
  Constant1 : Constant  Value=0.5*mb*g*Lr/(Lf+Lr)  OutDataTypeStr=single
  Constant2 : Constant  Value=0.5*mb*g*Lr/(Lf+Lr)+mw*g  OutDataTypeStr=single
  Gain : Gain  Gain=1/mw
  Gain1 : Gain  Gain=kw
  Gain2 : Gain  Gain=kw
  integrator1 : Subsystem
  integrator2 : Subsystem
  Fzs_fr : Outport  VectorParamsAs1DForOutWhenUnconnected=off
  Fzw_fr : Outport  Port=2  VectorParamsAs1DForOutWhenUnconnected=off
  wires:
  Add5/1 -> Fzs_fr/1
  Constant1/1 -> Add5/2
  Add3/1 -> Add4/2, Add5/1  "F2zs_fl"
  Gain/1 -> integrator1/1(In)
  Add4/1 -> Gain/1
  .1/1 -> Add3/2
  ./1 -> Add3/1
  Add2/1 -> .1/1
  dot_Zs_fr/1 -> Add2/2
  Add1/1 -> ./1
  Zs_fr/1 -> Add1/2
  Add/1 -> Gain1/1
  integrator2/1(Out) -> Add/1, Add1/1, Add6/2  "Zw_fl"
  integrator1/1(Out) -> integrator2/1(In), Add2/1
  Z_road_fr/1 -> Add6/1, Add/2
  Gain1/1 -> Add4/1  "F2zw_fl"
  Add6/1 -> Gain2/1
  Gain2/1 -> Add7/1  "F2zw_fl"
  Constant2/1 -> Add7/2
  Add7/1 -> Fzw_fr/1

== system VMC_14Dof_2024a/Subsystem/Body/Suspension_Z/integrator1 ==
  In : Inport
  Add : Sum
  Add1 : Sum
  Constant : Constant  Value=Sampletime  OutDataTypeStr=single
  Constant1 : Constant  Value=0  OutDataTypeStr=single
  Delay1 : Delay  DelayLength=1  InitialCondition=0
  Divide : Product  Inputs=**
  Out : Outport  VectorParamsAs1DForOutWhenUnconnected=off
  wires:
  In/1 -> Divide/1
  Constant/1 -> Divide/2
  Divide/1 -> Add/1
  Delay1/1 -> Add/2, Add1/2
  Constant1/1 -> Add1/1
  Add/1 -> Delay1/1
  Add1/1 -> Out/1

== system VMC_14Dof_2024a/Subsystem/Body/Suspension_Z/integrator2 ==
  In : Inport
  Add : Sum
  Add1 : Sum
  Constant : Constant  Value=Sampletime  OutDataTypeStr=single
  Constant1 : Constant  Value=0  OutDataTypeStr=single
  Delay1 : Delay  DelayLength=1  InitialCondition=0
  Divide : Product  Inputs=**
  Out : Outport  VectorParamsAs1DForOutWhenUnconnected=off
  wires:
  In/1 -> Divide/1
  Constant/1 -> Divide/2
  Divide/1 -> Add/1
  Delay1/1 -> Add/2, Add1/2
  Constant1/1 -> Add1/1
  Add/1 -> Delay1/1
  Add1/1 -> Out/1

== system VMC_14Dof_2024a/Subsystem/Body/Suspension_Z/integrator3 ==
  In : Inport
  Add : Sum
  Add1 : Sum
  Constant : Constant  Value=Sampletime  OutDataTypeStr=single
  Constant1 : Constant  Value=0  OutDataTypeStr=single
  Delay1 : Delay  DelayLength=1  InitialCondition=0
  Divide : Product  Inputs=**
  Out : Outport  VectorParamsAs1DForOutWhenUnconnected=off
  wires:
  In/1 -> Divide/1
  Constant/1 -> Divide/2
  Divide/1 -> Add/1
  Delay1/1 -> Add/2, Add1/2
  Constant1/1 -> Add1/1
  Add/1 -> Delay1/1
  Add1/1 -> Out/1

== system VMC_14Dof_2024a/Subsystem/Body/Suspension_Z/integrator7 ==
  In : Inport
  Add : Sum
  Add1 : Sum
  Constant : Constant  Value=Sampletime  OutDataTypeStr=single
  Constant1 : Constant  Value=0  OutDataTypeStr=single
  Delay1 : Delay  DelayLength=1  InitialCondition=0
  Divide : Product  Inputs=**
  Out : Outport  VectorParamsAs1DForOutWhenUnconnected=off
  wires:
  In/1 -> Divide/1
  Constant/1 -> Divide/2
  Divide/1 -> Add/1
  Delay1/1 -> Add/2, Add1/2
  Constant1/1 -> Add1/1
  Add/1 -> Delay1/1
  Add1/1 -> Out/1

== system VMC_14Dof_2024a/Subsystem/Body/Suspension_Z/rl ==
  dot_Zs_rl : Inport
  Z_road_rl : Inport  Port=2
  Zs_rl : Inport  Port=3
  . : Gain  Gain=ks_f
  .1 : Gain  Gain=Cs_f
  Add : Sum  Inputs=-+
  Add{1..2,4,6} (4 alike) : Sum  Inputs=+-
  Add3 : Sum
  Add5 : Sum
  Add7 : Sum  OutDataTypeStr=single
  Constant1 : Constant  Value=0.5*mb*g*Lf/(Lf+Lr)  OutDataTypeStr=single
  Constant2 : Constant  Value=0.5*mb*g*Lf/(Lf+Lr)+mw*g  OutDataTypeStr=single
  Gain : Gain  Gain=1/mw
  Gain1 : Gain  Gain=kw
  Gain2 : Gain  Gain=kw
  integrator1 : Subsystem
  integrator2 : Subsystem
  Fzs_rl : Outport  VectorParamsAs1DForOutWhenUnconnected=off
  Fzw_fl : Outport  Port=2  VectorParamsAs1DForOutWhenUnconnected=off
  wires:
  Add5/1 -> Fzs_rl/1
  Constant1/1 -> Add5/2
  Add3/1 -> Add4/2, Add5/1  "F2zs_fl"
  Gain/1 -> integrator1/1(In)
  Add4/1 -> Gain/1
  .1/1 -> Add3/2
  ./1 -> Add3/1
  Add2/1 -> .1/1
  dot_Zs_rl/1 -> Add2/2
  Add1/1 -> ./1
  Zs_rl/1 -> Add1/2
  Add/1 -> Gain1/1
  integrator2/1(Out) -> Add/1, Add1/1, Add6/2  "Zw_fl"
  integrator1/1(Out) -> integrator2/1(In), Add2/1
  Z_road_rl/1 -> Add6/1, Add/2
  Gain1/1 -> Add4/1  "F2zw_fl"
  Add6/1 -> Gain2/1
  Gain2/1 -> Add7/1  "F2zw_fl"
  Constant2/1 -> Add7/2
  Add7/1 -> Fzw_fl/1

== system VMC_14Dof_2024a/Subsystem/Body/Suspension_Z/rr ==
  dot_Zs_rr : Inport
  Z_road_rr : Inport  Port=2
  Zs_rr : Inport  Port=3
  . : Gain  Gain=ks_f
  .1 : Gain  Gain=Cs_f
  Add : Sum  Inputs=-+
  Add{1..2,4,6} (4 alike) : Sum  Inputs=+-
  Add3 : Sum
  Add5 : Sum
  Add7 : Sum  OutDataTypeStr=single
  Constant1 : Constant  Value=0.5*mb*g*Lf/(Lf+Lr)  OutDataTypeStr=single
  Constant2 : Constant  Value=0.5*mb*g*Lf/(Lf+Lr)+mw*g  OutDataTypeStr=single
  Gain : Gain  Gain=1/mw
  Gain1 : Gain  Gain=kw
  Gain2 : Gain  Gain=kw
  integrator1 : Subsystem
  integrator2 : Subsystem
  Fzs_rr : Outport  VectorParamsAs1DForOutWhenUnconnected=off
  Fzw_fl : Outport  Port=2  VectorParamsAs1DForOutWhenUnconnected=off
  wires:
  Add5/1 -> Fzs_rr/1
  Constant1/1 -> Add5/2
  Add3/1 -> Add4/2, Add5/1  "F2zs_fl"
  integrator1/1(Out) -> integrator2/1(In), Add2/1
  integrator2/1(Out) -> Add6/2, Add1/1, Add/1  "Zw_fl"
  Add/1 -> Gain1/1
  Zs_rr/1 -> Add1/2
  Add1/1 -> ./1
  dot_Zs_rr/1 -> Add2/2
  Add2/1 -> .1/1
  ./1 -> Add3/1
  .1/1 -> Add3/2
  Add4/1 -> Gain/1
  Gain/1 -> integrator1/1(In)
  Z_road_rr/1 -> Add6/1, Add/2
  Gain1/1 -> Add4/1  "F2zw_fl"
  Add6/1 -> Gain2/1
  Gain2/1 -> Add7/1  "F2zw_fl"
  Constant2/1 -> Add7/2
  Add7/1 -> Fzw_fl/1

== system VMC_14Dof_2024a/Subsystem/Body/Suspension_Z/zb_to_zs ==
  ddot_phi : Inport
  ddot_theta : Inport  Port=2
  ddot_zb : Inport  Port=3
  Bf/2 : Gain  Gain=0.5*Bf
  Br/2 : Gain  Gain=0.5*Br
  Lf : Gain  Gain=Lf
  Lr : Gain  Gain=Lr
  Sum1 : Sum  Inputs=+--
  Sum2 : Sum  Inputs=+++
  Sum3 : Sum  Inputs=+-+
  Sum8 : Sum  Inputs=++-
  integrator1 : Subsystem
  integrator2 : Subsystem
  integrator3 : Subsystem
  integrator7 : Subsystem
  dot_Zs_fl : Outport  VectorParamsAs1DForOutWhenUnconnected=off
  dot_Zs_fr : Outport  Port=2  VectorParamsAs1DForOutWhenUnconnected=off
  dot_Zs_rl : Outport  Port=3  VectorParamsAs1DForOutWhenUnconnected=off
  dot_Zs_rr : Outport  Port=4  VectorParamsAs1DForOutWhenUnconnected=off
  wires:
  ddot_phi/1 -> Br/2/1, Bf/2/1
  ddot_theta/1 -> Lr/1, Lf/1
  ddot_zb/1 -> Sum8/1, Sum1/1, Sum3/1, Sum2/1
  Bf/2/1 -> Sum1/2, Sum8/2
  Lf/1 -> Sum1/3, Sum8/3
  Sum8/1 -> integrator7/1(In)
  Sum1/1 -> integrator1/1(In)
  Br/2/1 -> Sum3/2, Sum2/2
  Lr/1 -> Sum3/3, Sum2/3
  Sum2/1 -> integrator3/1(In)
  Sum3/1 -> integrator2/1(In)
  integrator7/1(Out) -> dot_Zs_fl/1
  integrator1/1(Out) -> dot_Zs_fr/1
  integrator3/1(Out) -> dot_Zs_rl/1
  integrator2/1(Out) -> dot_Zs_rr/1

== system VMC_14Dof_2024a/Subsystem/Body/global system transform/integrator1 ==
  In : Inport
  Add : Sum
  Add1 : Sum
  Constant : Constant  Value=Sampletime  OutDataTypeStr=single
  Constant1 : Constant  Value=0  OutDataTypeStr=single
  Delay1 : Delay  DelayLength=1  InitialCondition=0
  Divide : Product  Inputs=**
  Out : Outport  VectorParamsAs1DForOutWhenUnconnected=off
  wires:
  In/1 -> Divide/1
  Constant/1 -> Divide/2
  Divide/1 -> Add/1
  Delay1/1 -> Add/2, Add1/2
  Constant1/1 -> Add1/1
  Add/1 -> Delay1/1
  Add1/1 -> Out/1
